simulink model "Inverted_Pendulum_FIX"  (R2015b)
settings: Solver=ode23t  SolverMode=SingleTasking  StartTime=0.0  StopTime=100  FixedStep=TS  MaxStep=TS  RelTol=1e-3
undefined symbols (not defined in the file): CONTROLLER_D, CONTROLLER_I, CONTROLLER_N, CONTROLLER_P, GRAVITY, INITIAL_POSITION, PENDULUM_FRICTION, PENDULUM_LENGTH, PENDULUM_MASS, PENDULUM_RADIUS, TORQUE_GAIN, TORQUE_LEVEL, TS, X, Y, Z
libraries: sm_lib x7, nesl_utility x5, State_Machine x3, simulink x1
settings Model: DataDictionary=Parameters.sldd  FPTRunName=FPA_Reference  PauseTimes=80  Creator=sdupertu  LastModifiedBy=sdupertu
settings DataIOCC: SaveFormat=Array
settings OptimizationCC: BlockReduction=off  DefaultParameterBehavior=Inlined  OptimizeModelRefInitCode=on  LifeSpan=1  MaxStackSize=64
settings DebuggingCC: SignalRangeChecking=warning  SaveWithParameterizedLinksMsg=none  SingleTaskRateTransMsg=error  ParameterDowncastMsg=warning  ParameterOverflowMsg=warning  ParameterPrecisionLossMsg=none  StrictBusMsg=ErrorOnBusTreatedAsVector
settings HardwareCC: ProdBitPerPointer=32  ProdLargestAtomicInteger=Long  ProdLargestAtomicFloat=Double  ProdIntDivRoundTo=Undefined  ProdWordSize=32  ProdHWDeviceType=ARM Compatible->ARM Cortex  TargetUnknown=on
settings RTWCC: SystemTargetFile=ert.tlc  TemplateMakefile=ert_default_tmf  Description=Embedded Coder  Toolchain=Xilinx Software Development Kit (SDK)
settings CodeAppCC: IgnoreCustomStorageClasses=off
settings ERTTargetCC: ERTCustomFileTemplate=example_file_process.tlc
settings ConfigComp: CovModelRefEnable=Off  CovSFcnEnable=off  PLC_TargetIDE=codesys23  PLC_ShowFullTargetList=off  PLC_GenerateReport=off

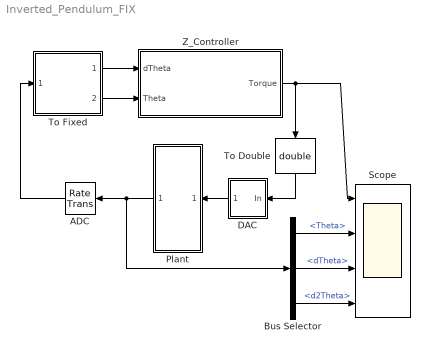
== system Inverted_Pendulum_FIX ==
  ADC : RateTransition  OutPortSampleTime=TS
  Bus Selector : BusSelector  OutputSignals=Theta,dTheta,d2Theta
  DAC : Subsystem  Variant=on  OverrideUsingVariant=DAC_ON
  Plant : Subsystem  Variant=on  OverrideUsingVariant=EQUATION
      settings: AttributesFormatString=%<BlockChoice>
      mask Display:
      | image('Pendulum.png');
      | % Get the active variant that has been selected
      | current_variant = get_param('Inverted_Pendulum_FIX/Plant','ActiveVariant');
      | % Reformat the text to avoid subscripts using the underscore character
      | displayed_name  = strrep(current_variant,'_',' ');
      | % Display the selected variant on the Simulink block
      | text(0.40,0.20,['{\fontsize{6pt}',displayed_name,'}'],...
      |      'texmode','on','hor','center','vert','middle','interpreter','tex');
  Scope : Scope  NumInputPorts=4
  To Double : DataTypeConversion  OutDataTypeStr=double
  To Fixed : Subsystem
  Z_Controller : Subsystem  MinMaxOverflowLogging=MinMaxAndOverflow  VariantControl=SIM_ROUND_Z
  wires:
  Plant/1(Measurements) -> Bus Selector/1, ADC/1
  Bus Selector/1 -> Scope/2  "<Theta>"
  Bus Selector/2 -> Scope/3  "<dTheta>"
  Bus Selector/3 -> Scope/4  "<d2Theta>"
  DAC/1(Out) -> Plant/1(Torque)
  To Double/1 -> DAC/1(In)
  ADC/1 -> To Fixed/1(Measurements)
  To Fixed/1(Theta_fixdt) -> Z_Controller/1(dTheta)
  To Fixed/2(dTheta_fixdt) -> Z_Controller/2(Theta)
  Z_Controller/1(Torque) -> To Double/1, Scope/1

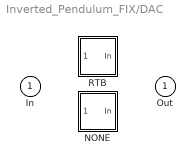
== system Inverted_Pendulum_FIX/DAC ==
  In : Inport
  NONE : Subsystem  VariantControl=DAC_OFF
  RTB : Subsystem  VariantControl=DAC_ON
  Out : Outport

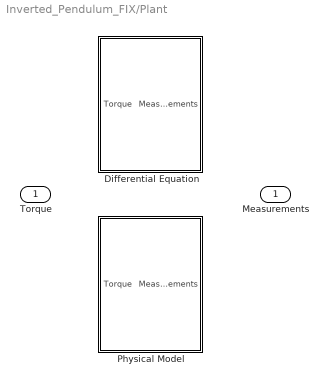
== system Inverted_Pendulum_FIX/Plant ==
  Torque : Inport
  Differential Equation : Subsystem  VariantControl=EQUATION  mask{Theta0=INITIAL_POSITION}
      mask prompts: Theta0 "Initial Position"
  Physical Model : Subsystem  VariantControl=PHYSICAL  mask{Theta0=INITIAL_POSITION}
      mask prompts: Theta0 "Initial Position"
  Measurements : Outport

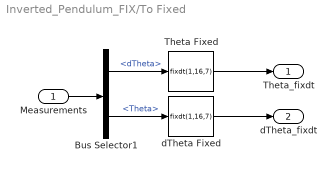
== system Inverted_Pendulum_FIX/To Fixed ==
  Measurements : Inport
  Bus Selector1 : BusSelector  OutputSignals=dTheta,Theta
  Theta Fixed : DataTypeConversion  OutMin=-2^8  OutMax=2^8-1  OutDataTypeStr=fixdt(1,16,7)
  dTheta Fixed : DataTypeConversion  OutMin=-2^8  OutMax=2^8-1  OutDataTypeStr=fixdt(1,16,7)
  Theta_fixdt : Outport
  dTheta_fixdt : Outport  Port=2
  wires:
  dTheta Fixed/1 -> dTheta_fixdt/1
  Measurements/1 -> Bus Selector1/1
  Bus Selector1/1 -> Theta Fixed/1  "<dTheta>"
  Bus Selector1/2 -> dTheta Fixed/1  "<Theta>"
  Theta Fixed/1 -> Theta_fixdt/1

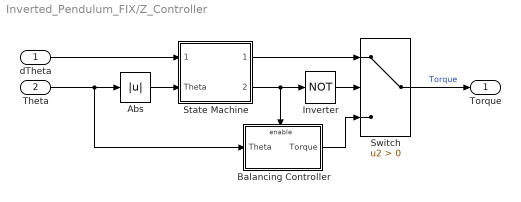
== system Inverted_Pendulum_FIX/Z_Controller ==
  dTheta : Inport  OutMin=-2^8  OutMax=2^8-1  OutDataTypeStr=fixdt(1,16,7)
  Theta : Inport  Port=2  OutMin=-2^8  OutMax=2^8-1  OutDataTypeStr=fixdt(1,16,7)
  Abs : Abs  OutDataTypeStr=fixdt(1,16,7)
  Balancing Controller : Subsystem  TreatAsAtomicUnit=on
  Inverter : Logic  Operator=NOT  AllPortsSameDT=off  OutDataTypeStr=boolean
  State Machine : Subsystem  Variant=on  OverrideUsingVariant=FIXED_PRECISION
      mask Display: image('State_Machine_Diagram.png');
  Switch : Switch  Criteria=u2 > Threshold  OutDataTypeStr=fixdt(1,16,7)
  Torque : Outport
  wires:
  Balancing Controller/1(Torque) -> Switch/3
  Inverter/1 -> Switch/2
  State Machine/2(Trigger) -> Balancing Controller/Enable, Inverter/1
  dTheta/1 -> State Machine/1(dTheta)
  State Machine/1(Torque) -> Switch/1
  Switch/1 -> Torque/1  "Torque"
  Abs/1 -> State Machine/2(Theta)
  Theta/1 -> Balancing Controller/1(Theta), Abs/1

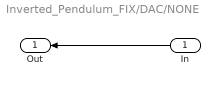
== system Inverted_Pendulum_FIX/DAC/NONE ==
  In : Inport
  Out : Outport
  wires:
  In/1 -> Out/1

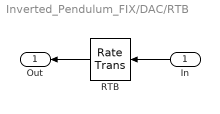
== system Inverted_Pendulum_FIX/DAC/RTB ==
  In : Inport
  RTB : RateTransition
  Out : Outport
  wires:
  RTB/1 -> Out/1
  In/1 -> RTB/1

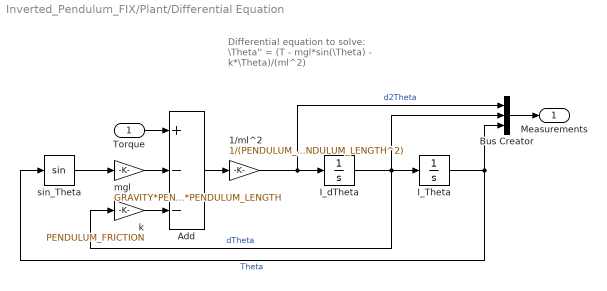
== system Inverted_Pendulum_FIX/Plant/Differential Equation ==
  note: Differential equation to solve:
      | \Theta'' = (T - mgl*sin(\Theta) - k*\Theta)/(ml^2)
  Torque : Inport
  1/ml^2 : Gain  Gain=1/(PENDULUM_MASS*PENDULUM_LENGTH^2)
  Add : Sum  Inputs=+--
  Bus Creator : BusCreator  Inputs=3
  I_Theta : Integrator  InitialCondition=Theta0
  I_dTheta : Integrator
  k : Gain  Gain=PENDULUM_FRICTION
  mgl : Gain  Gain=GRAVITY*PENDULUM_MASS*PENDULUM_LENGTH
  sin_Theta : Trigonometry
  Measurements : Outport
  wires:
  Bus Creator/1 -> Measurements/1
  mgl/1 -> Add/2
  Torque/1 -> Add/1
  Add/1 -> 1/ml^2/1
  sin_Theta/1 -> mgl/1
  I_dTheta/1 -> k/1, Bus Creator/2, I_Theta/1  "dTheta"
  I_Theta/1 -> Bus Creator/3, sin_Theta/1  "Theta"
  1/ml^2/1 -> Bus Creator/1, I_dTheta/1  "d2Theta"
  k/1 -> Add/3

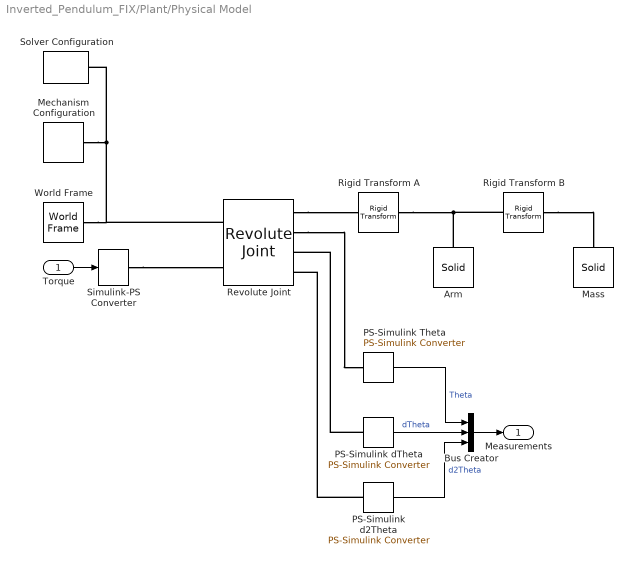
== system Inverted_Pendulum_FIX/Plant/Physical Model ==
  Torque : Inport
  Arm : sm_lib/Body Elements/Solid  InertiaType=CalculateFromGeometry  Mass=1  MassUnits=kg  CenterOfMass=[0 0 0]  CenterOfMassUnits=m  MomentsOfInertia=[1 1 1]  MomentsOfInertiaUnits=kg*m^2  ProductsOfInertia=[0 0 0]  ProductsOfInertiaUnits=kg*m^2  DensityBased=on  Density=0.001  DensityUnits=kg/(m^3)  GraphicType=FromGeometry  MarkerShape=Sphere  MarkerSize=10  MarkerSizeUnits=m  GraphicVisPropType=SimpleVisualProperties  GraphicDiffuseColor=[0 0 0]  GraphicSpecularColor=[0.5 0.5 0.5 1.0]  GraphicAmbientColor=[0.15 0.15 0.15 1.0]  GraphicEmissiveColor=[0.0 0.0 0.0 1.0]  GraphicShininess=75  GraphicOpacity=1.0  GeometryShape=Brick  RectangleSize=[1 1]  RectangleSizeUnits=m  BrickDimensions=[0.01 PENDULUM_LENGTH 0.01]  BrickDimensionUnits=m  CylinderRadius=1  CylinderRadiusUnits=m  CylinderLength=1  CylinderLengthUnits=m  SphereRadius=1  SphereRadiusUnits=m  EllipsoidRadii=[1 1 1]  EllipsoidRadiiUnits=m  ExtrusionCrossSection=[1 1; -1 1; -1 -1; 1 -1]  ExtrusionCrossSectionUnits=m  ExtrusionLength=1  ExtrusionLengthUnits=m  PolygonNumSides=3  PolygonOuterRadius=1  PolygonOuterRadiusUnits=m  ExtGeomFileType=STL  ExtGeomFileUnits=m  RevolutionCrossSection=[1 1; 1 -1; 2 -1; 2 1]  RevolutionCrossSectionUnits=m  RevolutionExtent=Full  RevolutionAngle=180  RevolutionAngleUnits=deg  BlockFunction=simmechanics.library.body_elements.solid
  Bus Creator : BusCreator  Inputs=3
  Mass : sm_lib/Body Elements/Solid  InertiaType=PointMass  Mass=PENDULUM_MASS  MassUnits=kg  CenterOfMass=[0 0 0]  CenterOfMassUnits=m  MomentsOfInertia=[1 1 1]  MomentsOfInertiaUnits=kg*m^2  ProductsOfInertia=[0 0 0]  ProductsOfInertiaUnits=kg*m^2  DensityBased=on  Density=1000  DensityUnits=kg/(m^3)  GraphicType=FromGeometry  MarkerShape=Sphere  MarkerSize=10  MarkerSizeUnits=m  GraphicVisPropType=SimpleVisualProperties  GraphicDiffuseColor=[1 0.5 0]  GraphicSpecularColor=[0.5 0.5 0.5 1.0]  GraphicAmbientColor=[0.15 0.15 0.15 1.0]  GraphicEmissiveColor=[0.0 0.0 0.0 1.0]  GraphicShininess=75  GraphicOpacity=1.0  GeometryShape=Sphere  RectangleSize=[1 1]  RectangleSizeUnits=m  BrickDimensions=[1 1 1]  BrickDimensionUnits=m  CylinderRadius=1  CylinderRadiusUnits=m  CylinderLength=1  CylinderLengthUnits=m  SphereRadius=PENDULUM_RADIUS  SphereRadiusUnits=m  EllipsoidRadii=[1 1 1]  EllipsoidRadiiUnits=m  ExtrusionCrossSection=[1 1; -1 1; -1 -1; 1 -1]  ExtrusionCrossSectionUnits=m  ExtrusionLength=1  ExtrusionLengthUnits=m  PolygonNumSides=3  PolygonOuterRadius=1  PolygonOuterRadiusUnits=m  ExtGeomFileType=STL  ExtGeomFileUnits=m  RevolutionCrossSection=[1 1; 1 -1; 2 -1; 2 1]  RevolutionCrossSectionUnits=m  RevolutionExtent=Full  RevolutionAngle=180  RevolutionAngleUnits=deg  BlockFunction=simmechanics.library.body_elements.solid
  Mechanism Configuration : sm_lib/Utilities/Mechanism Configuration  UniformGravity=Constant  GravityVector=[0 GRAVITY 0]  GravityUnits=m/s^2  LinearizationDelta=0.001  BlockFunction=simmechanics.library.utilities.mechanism_configuration
  PS-Simulink Theta : nesl_utility/PS-Simulink Converter  PhysicalDomain=network_engine_domain  SubClassName=ps_output  LeftPortType=input  RightPortType=output  PseudoPeriodic=off  Frequencies=[]  Unit=rad  AffineConversion=off
  PS-Simulink d2Theta : nesl_utility/PS-Simulink Converter  PhysicalDomain=network_engine_domain  SubClassName=ps_output  LeftPortType=input  RightPortType=output  PseudoPeriodic=off  Frequencies=[]  Unit=rad/s^2  AffineConversion=off
  PS-Simulink dTheta : nesl_utility/PS-Simulink Converter  PhysicalDomain=network_engine_domain  SubClassName=ps_output  LeftPortType=input  RightPortType=output  PseudoPeriodic=off  Frequencies=[]  Unit=rad/s  AffineConversion=off
  Revolute Joint : sm_lib/Joints/Revolute Joint  SenseConstraintForce=off  SenseConstraintForceX=off  SenseConstraintForceY=off  SenseConstraintForceZ=off  SenseConstraintTorque=off  SenseConstraintTorqueX=off  SenseConstraintTorqueY=off  SenseConstraintTorqueZ=off  SenseTotalForce=off  SenseTotalForceX=off  SenseTotalForceY=off  SenseTotalForceZ=off  SenseTotalTorque=off  SenseTotalTorqueX=off  SenseTotalTorqueY=off  SenseTotalTorqueZ=off  CompositeWrenchDir=FollowerOnBase  CompositeWrenchFrame=BaseFrame  EquilibriumPosition=0  EquilibriumPositionUnits=rad  SpringStiffness=0  SpringStiffnessUnits=N*m/deg  DampingCoefficient=PENDULUM_FRICTION  DampingCoefficientUnits=N*m/(rad/s)  TorqueActuationMode=InputTorque  MotionActuationMode=ComputedMotion  SensePosition=on  SenseVelocity=on  SenseAcceleration=on  SenseTorqueForce=off  PositionTargetSpecify=on  PositionTargetPriority=High  PositionTargetValue=-pi  PositionTargetValueUnits=rad  VelocityTargetSpecify=on  VelocityTargetPriority=High  VelocityTargetValue=0  VelocityTargetValueUnits=rad/s  BlockFunction=simmechanics.library.joints.revolute_joint
  Rigid Transform A : sm_lib/Frames and Transforms/Rigid Transform  TranslationMethod=StandardAxis  TranslationLengthUnit=m  TranslationStandardAxis=+Y  TranslationStandardOffset=PENDULUM_LENGTH/2  TranslationCartesianOffset=[0 0 0]  TranslationROffset=0  TranslationROffsetUnits=m  TranslationZOffset=0  TranslationZOffsetUnits=m  TranslationThetaOffset=0  TranslationThetaOffsetUnits=deg  RotationMethod=None  RotationAngleUnits=deg  RotationStandardAxis=+Z  RotationAngle=0.0  RotationArbitraryAxis=[0 0 1]  FollAlignAxisA=+X  BaseAlignAxisA=+Y  FollAlignAxisB=+Y  BaseAlignAxisB=+Z  RotationMatrix=[1 0 0; 0 1 0; 0 0 1]  BlockFunction=simmechanics.library.frames_transforms.rigid_transform
  Rigid Transform B : sm_lib/Frames and Transforms/Rigid Transform  TranslationMethod=StandardAxis  TranslationLengthUnit=m  TranslationStandardAxis=+Y  TranslationStandardOffset=PENDULUM_LENGTH/2+PENDULUM_RADIUS  TranslationCartesianOffset=[0 0 0]  TranslationROffset=0  TranslationROffsetUnits=m  TranslationZOffset=0  TranslationZOffsetUnits=m  TranslationThetaOffset=0  TranslationThetaOffsetUnits=deg  RotationMethod=None  RotationAngleUnits=deg  RotationStandardAxis=+Z  RotationAngle=0.0  RotationArbitraryAxis=[0 0 1]  FollAlignAxisA=+X  BaseAlignAxisA=+Y  FollAlignAxisB=+Y  BaseAlignAxisB=+Z  RotationMatrix=[1 0 0; 0 1 0; 0 0 1]  BlockFunction=simmechanics.library.frames_transforms.rigid_transform
  Simulink-PS Converter : nesl_utility/Simulink-PS Converter  PhysicalDomain=network_engine_domain  SubClassName=ps_input  LeftPortType=input  RightPortType=output  PseudoPeriodic=off  Frequencies=[]  NoiseDistribution=none  NoiseParameters=[]  Unit=N*m  AffineConversion=off  InputFiltering=on  SimscapeFilterOrder=2  InputFilterTimeConstant=0.001  UdotUserProvided=1
  Solver Configuration : nesl_utility/Solver Configuration  PhysicalDomain=network_engine_domain  SubClassName=solver  LeftPortType=input  RightPortType=generic  Accelerate=off  Tones=[]  Harmonics=[]  SimulateNoise=off  Profile=off  UseLocalSampling=off  EnableSwitchedLinearOptims=on  FrequencyDomain=off  UseCCode=off  RelTol=0.001  AbsTol=1e-06  MinStep=1e-09  ToWorkspace=off  RevertToSquareIcSolve=off  NumHomotopyIterations=100  DoDC=off  ResidualTolerance=1e-09  UseLocalSolver=off  LocalSolverChoice=NE_TRAPEZOIDAL_ADVANCER  LocalSolverSampleTime=0.0001  DoFixedCost=off  MaxNonlinIter=3  MaxModeIter=2  LinearAlgebra=Sparse  DelaysMemoryBudget=1024  AutomaticFiltering=on  FilteringTimeConstant=0.001
  World Frame : sm_lib/Frames and Transforms/World Frame  BlockFunction=simmechanics.library.frames_transforms.world_frame
  Measurements : Outport
  wires:
  Bus Creator/1 -> Measurements/1
  Torque/1 -> Simulink-PS Converter/1
  PS-Simulink dTheta/1 -> Bus Creator/2  "dTheta"
  PS-Simulink d2Theta/1 -> Bus Creator/3  "d2Theta"
  PS-Simulink Theta/1 -> Bus Creator/1  "Theta"
  connections:
  Mechanism Configuration/RConn1 -- World Frame/RConn1 -- Revolute Joint/LConn1 -- Solver Configuration/RConn1
  Rigid Transform A/RConn1 -- Arm/RConn1 -- Rigid Transform B/LConn1
  Revolute Joint/RConn1 -- Rigid Transform A/LConn1
  Rigid Transform B/RConn1 -- Mass/RConn1
  Simulink-PS Converter/RConn1 -- Revolute Joint/LConn2
  PS-Simulink dTheta/LConn1 -- Revolute Joint/RConn3
  PS-Simulink d2Theta/LConn1 -- Revolute Joint/RConn4
  Revolute Joint/RConn2 -- PS-Simulink Theta/LConn1

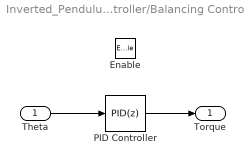
== system Inverted_Pendulum_FIX/Z_Controller/Balancing Controller ==
  Theta : Inport
  Enable : EnablePort
  PID Controller : simulink/Continuous/PID Controller  Controller=PID  TimeDomain=Discrete-time  SampleTime=TS  IntegratorMethod=Forward Euler  FilterMethod=Forward Euler  Form=Parallel  UseFilter=on  ControllerParametersSource=internal  P=CONTROLLER_P  I=CONTROLLER_I  D=CONTROLLER_D  N=CONTROLLER_N  InitialConditionSource=internal  InitialConditionForIntegrator=0  InitialConditionForFilter=0  ExternalReset=none  LimitOutput=on  UpperSaturationLimit=TORQUE_LEVEL*TORQUE_GAIN  LowerSaturationLimit=-TORQUE_LEVEL*TORQUE_GAIN  LinearizeAsGain=off  AntiWindupMode=back-calculation  Kb=1  TrackingMode=off  Kt=1  PParamMin=[]  PParamMax=[]  PParamDataTypeStr=fixdt(1,16,7)  IParamMin=[]  IParamMax=[]  IParamDataTypeStr=fixdt(1,16,7)  DParamMin=[]  DParamMax=[]  DParamDataTypeStr=fixdt(1,16,7)  NParamMin=[]  NParamMax=[]  NParamDataTypeStr=fixdt(1,16,7)  KbParamMin=[]  KbParamMax=[]  KbParamDataTypeStr=fixdt(1,16,7)  KtParamMin=[]  KtParamMax=[]  POutMin=[]  POutMax=[]  POutDataTypeStr=fixdt(1,16,7)  PGainOutDataTypeStr=fixdt(1,16,7)  PProdOutDataTypeStr=fixdt(1,16,7)  IOutMin=[]  IOutMax=[]  IOutDataTypeStr=fixdt(1,16,7)  IGainOutDataTypeStr=fixdt(1,16,7)  IProdOutDataTypeStr=fixdt(1,16,7)  DOutMin=[]  DOutMax=[]  DOutDataTypeStr=fixdt(1,16,7)  DGainOutDataTypeStr=fixdt(1,16,7)  DProdOutDataTypeStr=fixdt(1,16,7)  NOutMin=[]  NOutMax=[]  NOutDataTypeStr=fixdt(1,16,7)  NGainOutDataTypeStr=fixdt(1,16,7)  NProdOutDataTypeStr=fixdt(1,16,7)  KbOutMin=[]  KbOutMax=[]  KbOutDataTypeStr=fixdt(1,16,7)  KtOutMin=[]  KtOutMax=[]  IntegratorOutMin=[]  IntegratorOutMax=[]  IntegratorOutDataTypeStr=fixdt(1,16,7)  FilterOutMin=[]  FilterOutMax=[]  FilterOutDataTypeStr=fixdt(1,16,7)  SumOutMin=[]  SumOutMax=[]  SumOutDataTypeStr=fixdt(1,16,7)  SumI1OutMin=[]  SumI1OutMax=[]  SumI1OutDataTypeStr=fixdt(1,16,7)  SumI2OutMin=[]  SumI2OutMax=[]  SumI2OutDataTypeStr=fixdt(1,16,7)  SumI3OutMin=[]  SumI3OutMax=[]  SumDOutMin=[]  SumDOutMax=[]  SumDOutDataTypeStr=fixdt(1,16,7)  SumAccumDataTypeStr=fixdt(1,16,7)  SumI1AccumDataTypeStr=fixdt(1,16,7)  SumI2AccumDataTypeStr=fixdt(1,16,7)  SumDAccumDataTypeStr=fixdt(1,16,7)  SaturationOutMin=[]  SaturationOutMax=[]  SaturationOutDataTypeStr=fixdt(1,16,7)  IntegratorContinuousStateAttributes=''  IntegratorStateMustResolveToSignalObject=off  IntegratorRTWStateStorageClass=Auto  FilterContinuousStateAttributes=''  FilterStateMustResolveToSignalObject=off  FilterRTWStateStorageClass=Auto  DifferentiatorICPrevScaledInput=0  DifferentiatorOutMin=[]  DifferentiatorOutMax=[]
      settings: LockScale=on
  Torque : Outport  InitialOutput=0
  wires:
  Theta/1 -> PID Controller/1
  PID Controller/1 -> Torque/1

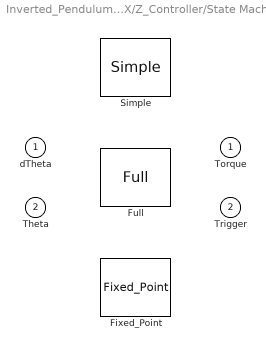
== system Inverted_Pendulum_FIX/Z_Controller/State Machine ==
  dTheta : Inport
  Theta : Inport  Port=2
  Fixed_Point : State_Machine/Fixed_Point  SystemSampleTime=-1  VariantControl=FIXED_PRECISION
  Full : State_Machine/Full  SystemSampleTime=-1  VariantControl=DOUBLE_PRECISION
  Simple : State_Machine/Simple  SystemSampleTime=-1  VariantControl=SIMPLE
  Torque : Outport
  Trigger : Outport  Port=2
